simulink model "task_3_scheme"  (R2024a)
settings: Solver=FixedStepAuto  StartTime=0.0  StopTime=10.0  FixedStep=0.001  RelTol=1e-3
settings Model: Creator=alexe  LastModifiedBy=alexe

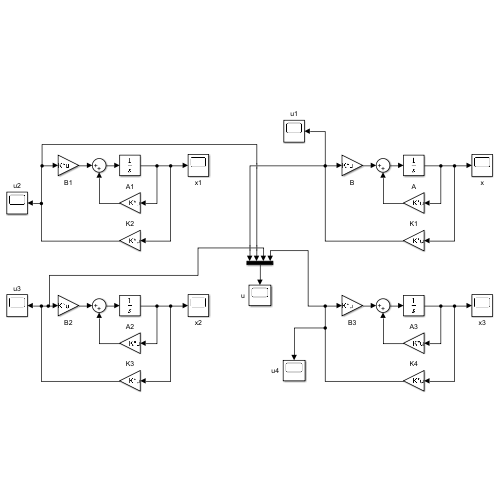
[thumbnail: Simulink's stored preview of the top-level diagram]
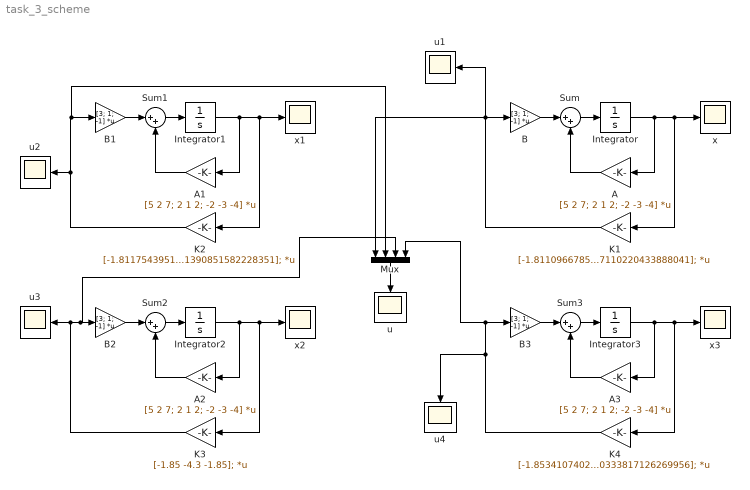
== system task_3_scheme ==
  A{,1..3} (4 alike) : Gain  Gain=[5 2 7; 2 1 2; -2 -3 -4]  Multiplication=Matrix(K*u)
  B{,1..3} (4 alike) : Gain  Gain=[3; 1; -1]  Multiplication=Matrix(K*u)
  Integrator{,1..3} (4 alike) : Integrator  InitialCondition=[1;1;1]
  K1 : Gain  Gain=[-1.8110966785064287110220433888041 -4.3160849593283698027780387510567 -1.8110966785064287110220433888041];  Multiplication=Matrix(K*u)
  K2 : Gain  Gain=[-1.8117543951362541390851582228351 -4.3177192340462210264038924401546 -1.8117543951362541390851582228351];  Multiplication=Matrix(K*u)
  K3 : Gain  Gain=[-1.85 -4.3 -1.85];  Multiplication=Matrix(K*u)
  K4 : Gain  Gain=[-1.8534107402031930333817126269956 -4.0261248185776487663280116110305 -1.8534107402031930333817126269956];  Multiplication=Matrix(K*u)
  Mux : Mux
  Sum{,1..3} (4 alike) : Sum  Inputs=|++
  u{,1..4} (5 alike) : Scope
  x{,1..3} (4 alike) : Scope
  wires:
  B/1 -> Sum/1
  Sum/1 -> Integrator/1
  A/1 -> Sum/2
  Integrator/1 -> A/1, K1/1, x/1
  K1/1 -> u1/1, Mux/1, B/1
  Integrator1/1 -> A1/1, K2/1, x1/1
  B1/1 -> Sum1/1
  Sum1/1 -> Integrator1/1
  A1/1 -> Sum1/2
  K2/1 -> Mux/2, B1/1, u2/1
  Integrator2/1 -> A2/1, K3/1, x2/1
  B2/1 -> Sum2/1
  Sum2/1 -> Integrator2/1
  A2/1 -> Sum2/2
  K3/1 -> u3/1, Mux/3, B2/1
  Integrator3/1 -> A3/1, K4/1, x3/1
  B3/1 -> Sum3/1
  Sum3/1 -> Integrator3/1
  A3/1 -> Sum3/2
  K4/1 -> u4/1, Mux/4, B3/1
  Mux/1 -> u/1
